simulink model "Lab2_model"  (R2023a)
settings: Solver=FixedStepAuto  StartTime=0.0  StopTime=0.5  FixedStep=0.00001  RelTol=1e-3
libraries: spsUniversalBridgeLib x2, spsAsynchronousMachineSIUnitsLib x1, simulink x1, spsCurrentMeasurementLib x1, spsSeriesRLCBranchLib x1, spsThreePhaseProgrammableVoltageSourceLib x1, spsVoltageMeasurementLib x1, sps_lib x1
settings Model: Creator=朱子轩  LastModifiedBy=Administrator

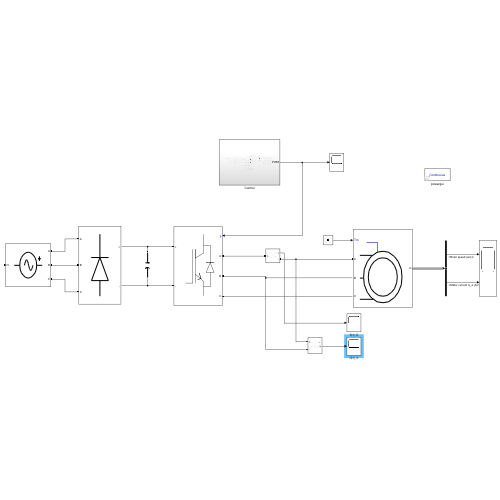
[thumbnail: Simulink's stored preview of the top-level diagram]
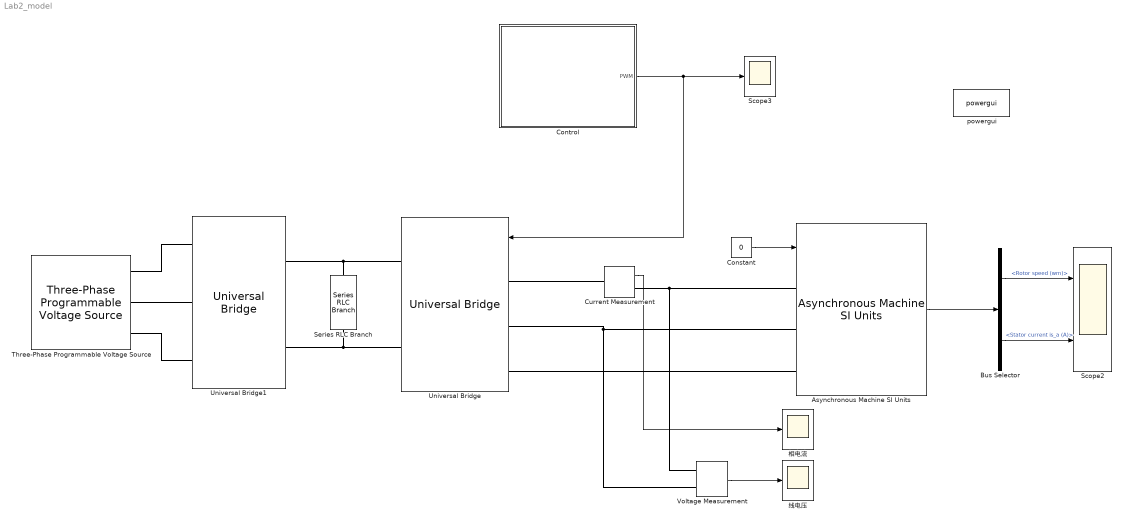
== system Lab2_model ==
  Asynchronous Machine SI Units : spsAsynchronousMachineSIUnitsLib/Asynchronous Machine SI Units  RotorType=Squirrel-cage  PresetModel="15:  5.4 HP (4KW)   400 V  50Hz 1430 RPM"  MechanicalLoad=Torque Tm  ShowDetailedParameters=on  ReferenceFrame=Rotor  Units=SI  MeasurementBus=off  NominalParameters=[4000 400 50]  VoltageRatio=1  Stator=[1.405 0.005839]  Rotor=[1.395 0.005839]  Cage1=[0.4155 0.002066]  Cage2=[0.4168 0.0003495]  Lm=0.1722  Mechanical=[0.0131 0.002985 2]  PolePairs=2  InitialConditions=[0 0 0 0 0 0 0 0]  SimulateSaturation=off  Saturation=[14.03593122, 27.81365428, 53.79336849, 72.68890987, 97.98006896, 148.6815601, 215.7428561, 302.9841135, 428.7778367 ; 230, 322, 414, 460, 506, 552, 598, 644, 690]  LoadFlowParameters=1492000  TsPowergui=0  TsBlock=-1  IterativeModel=Trapezoidal non iterative  IterativeDiscreteModel=Trapezoidal non iterative  Pmec=1.492e+006
  Bus Selector : BusSelector  OutputSignals=Mechanical.Rotor speed (wm),Stator measurements.Stator current is_a (A)
  Constant : Constant  Value=0
  Control : Subsystem
  Current Measurement : spsCurrentMeasurementLib/Current Measurement  PhasorSimulation=off  OutputType=Complex  PSBequivalent=0
  Scope2 : Scope  NumInputPorts=2
  Scope3 : Scope
  Series RLC Branch : spsSeriesRLCBranchLib/Series RLC Branch  LConnTagsString=__new0  RConnTagsString=__new0  BranchType=C  Resistance=0  Inductance=1e-3  SetiL0=off  InitialCurrent=0  Capacitance=1e-3  Setx0=off  InitialVoltage=0  Measurements=None
  Three-Phase Programmable Voltage Source : spsThreePhaseProgrammableVoltageSourceLib/Three-Phase Programmable Voltage Source  PositiveSequence=[380 0 50]  VariationEntity=None  VariationType=Table of time-amplitude pairs  VariationTypeAlt=Step  VariationStep=0.5  VariationRate=10  VariationMagnitude=0.3  VariationFrequency=2  VariationTiming=[1 2]  VariationPhaseA=off  Amplitudes=[1 0.8 1.2 1.0]  TimeValues=[0 0.1 0.15 0.2]  HarmonicGeneration=off  HarmonicA=[3 0.2 -25 0]  HarmonicB=[2 0.15 35 2]  Timing="[0.05  3]"  BusType=swing  Pref=0  Qref=0  Qmin=-inf  Qmax=inf
  Universal Bridge : spsUniversalBridgeLib/Universal Bridge  Arms=3  SnubberResistance=1e5  SnubberCapacitance=1e-9  Device=IGBT / Diodes  Ron=1e-3  Lon=0  ForwardVoltages="[  0  0  ]"  ForwardVoltage=0  GTOparameters=[ 10e-6 , 20e-6 ]  IGBTparameters=[ 1e-6 , 2e-6 ]  Measurements=None  Measurements_2=None  converterType=Rectifier
  Universal Bridge1 : spsUniversalBridgeLib/Universal Bridge  Arms=3  SnubberResistance=1e5  SnubberCapacitance=1e-9  Device=Diodes  Ron=1e-3  Lon=0  ForwardVoltages="[  0  0  ]"  ForwardVoltage=0  GTOparameters=[ 10e-6 , 20e-6 ]  IGBTparameters=[ 1e-6 , 2e-6 ]  Measurements=None  Measurements_2=None  converterType=Rectifier
  Voltage Measurement : spsVoltageMeasurementLib/Voltage Measurement  PhasorSimulation=off  OutputType=Complex  PSBequivalent=0
  powergui : sps_lib/powergui  Priority=1  SimulationMode=Continuous  SampleTime=5e-06  frequency=60  Iterations=50  frequencyindice=50  Pbase=100e6  ErrMax=1e-4  UnitsV=kV  UnitsW=MW  buscounter=0  FunctionMessages=off  echomessages=off  EnableUseOfTLC=off  CurrentSourceSwitches=off  DisableSnubberDevices=off  DisableRonSwitches=off  DisableVfSwitches=off  DisplayEquations=off  AutomaticDiscreteSolvers=off  SolverType=Tustin/Backward Euler (TBE)  Interpol=off  ExternalGateDelay=off  methode=off  Ts=100  x0status=blocks  SPID=on  SwTol=0  HookPort=off  NonlinearTolerance=1e-4  nMaxIteration=100  ContinueOnMaxIteration=off  RestoreLinks=warning  ResistiveCurrentMeasurement=off  Frange=[0:2:500]  Ylog=off  Xlog=on  ShowGrid=off  save=off  variable=ZData  structure=0  ZoomFFT=off  StartTime=0.0  cycles=1  DisplayStyle=1  fundamental=60  FreqAxis=off  MaxFrequency=1000  frequencyindicesteady=1  RmsSteady=1  display=off
  相电流 : Scope
  线电压 : Scope
  wires:
  Voltage Measurement/1 -> 线电压/1
  Current Measurement/1 -> 相电流/1
  Constant/1 -> Asynchronous Machine SI Units/1
  Asynchronous Machine SI Units/1 -> Bus Selector/1
  Bus Selector/1 -> Scope2/1  "<Rotor speed (wm)>"
  Bus Selector/2 -> Scope2/2  "<Stator current is_a (A)>"
  Control/1(PWM) -> Universal Bridge/1, Scope3/1
  connections:
  Three-Phase Programmable Voltage Source/RConn2 -- Universal Bridge1/LConn2
  Three-Phase Programmable Voltage Source/RConn1 -- Universal Bridge1/LConn1
  Three-Phase Programmable Voltage Source/RConn3 -- Universal Bridge1/LConn3
  Universal Bridge1/RConn1 -- Universal Bridge/RConn1 -- Series RLC Branch/LConn1
  Universal Bridge1/RConn2 -- Universal Bridge/RConn2 -- Series RLC Branch/RConn1
  Current Measurement/RConn1 -- Voltage Measurement/LConn1 -- Asynchronous Machine SI Units/LConn1
  Universal Bridge/LConn1 -- Current Measurement/LConn1
  Universal Bridge/LConn2 -- Voltage Measurement/LConn2 -- Asynchronous Machine SI Units/LConn2
  Universal Bridge/LConn3 -- Asynchronous Machine SI Units/LConn3

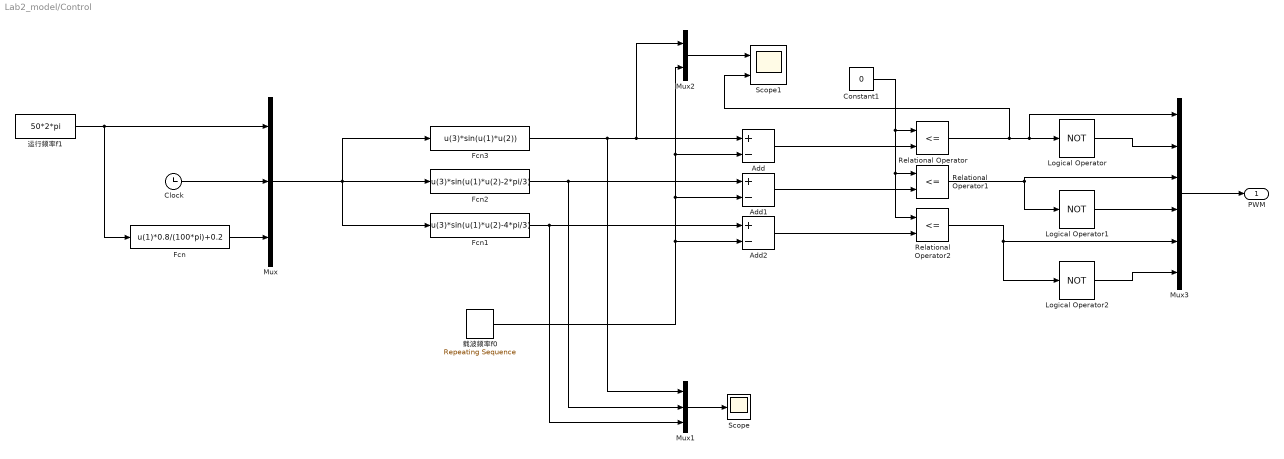
== system Lab2_model/Control ==
  Add : Sum  Inputs=+-
  Add1 : Sum  Inputs=+-
  Add2 : Sum  Inputs=+-
  Clock : Clock
  Constant1 : Constant  Value=0
  Fcn : Fcn  Expr=u(1)*0.8/(100*pi)+0.2
  Fcn1 : Fcn  Expr=u(3)*sin(u(1)*u(2)-4*pi/3)
  Fcn2 : Fcn  Expr=u(3)*sin(u(1)*u(2)-2*pi/3)
  Fcn3 : Fcn  Expr=u(3)*sin(u(1)*u(2))
  Logical Operator : Logic  Operator=NOT  AllPortsSameDT=off  OutDataTypeStr=boolean
  Logical Operator1 : Logic  Operator=NOT  AllPortsSameDT=off  OutDataTypeStr=boolean
  Logical Operator2 : Logic  Operator=NOT  AllPortsSameDT=off  OutDataTypeStr=boolean
  Mux : Mux  Inputs=3
  Mux1 : Mux  Inputs=3
  Mux2 : Mux  Inputs=2
  Mux3 : Mux  Inputs=6
  Relational Operator : RelationalOperator  Operator=<=  OutDataTypeStr=boolean  RndMeth=Simplest  InputSameDT=off
  Relational Operator1 : RelationalOperator  Operator=<=  OutDataTypeStr=boolean  RndMeth=Simplest  InputSameDT=off
  Relational Operator2 : RelationalOperator  Operator=<=  OutDataTypeStr=boolean  RndMeth=Simplest  InputSameDT=off
  Scope : Scope
  Scope1 : Scope  NumInputPorts=2
  载波频率f0 : simulink/Sources/Repeating Sequence  rep_seq_t=[0 1/3000 1/1500]  rep_seq_y=[-1 1 -1]
  运行频率f1 : Constant  Value=50*2*pi
  PWM : Outport
  wires:
  运行频率f1/1 -> Fcn/1, Mux/1
  Clock/1 -> Mux/2
  Fcn/1 -> Mux/3
  Mux/1 -> Fcn1/1, Fcn2/1, Fcn3/1
  Fcn3/1 -> Mux1/1, Mux2/1, Add/1
  Fcn2/1 -> Add1/1, Mux1/2
  Fcn1/1 -> Add2/1, Mux1/3
  Mux1/1 -> Scope/1
  载波频率f0/1 -> Add2/2, Add1/2, Mux2/2, Add/2
  Mux2/1 -> Scope1/1
  Add/1 -> Relational Operator/2
  Add2/1 -> Relational Operator2/2
  Add1/1 -> Relational Operator1/2
  Constant1/1 -> Relational Operator2/1, Relational Operator1/1, Relational Operator/1
  Relational Operator/1 -> Scope1/2, Mux3/1, Logical Operator/1
  Relational Operator1/1 -> Mux3/3, Logical Operator1/1
  Relational Operator2/1 -> Logical Operator2/1, Mux3/5
  Logical Operator/1 -> Mux3/2
  Logical Operator1/1 -> Mux3/4
  Logical Operator2/1 -> Mux3/6
  Mux3/1 -> PWM/1
